simulink model "simulation_UMFCBF_"  (R2022a)
settings: Solver=VariableStepAuto  StartTime=0.0  StopTime=simTime  RelTol=1e-3
values from neighbouring files (symbols this model uses):
  a = 0.1    [setup_UMFCBF.m]
  delta = 2    [setup_UMFCBF.m]
  Icm = 1/2*m*robot_radius^2    (= 0.2385)    [setup_UMFCBF.m]
  Kd = 2.7    [setup_UMFCBF.m]
  Kp = 0.1    [setup_UMFCBF.m]
  m = 5.3    [setup_UMFCBF.m]
  obstacles = setup_environment(MAP,a,robot_radius)    [setup_UMFCBF.m]
  qg = [8 ; -3]    [setup_UMFCBF.m]
  qstart = [0 0 pi/2]'    [setup_UMFCBF.m]
  threshold_skip = 0    [setup_UMFCBF.m]
  vwstart = [0 0]'    [setup_UMFCBF.m]
libraries: slctrlblks x1
settings Model: Creator=mirkomizzoni  LastModifiedBy=dennis

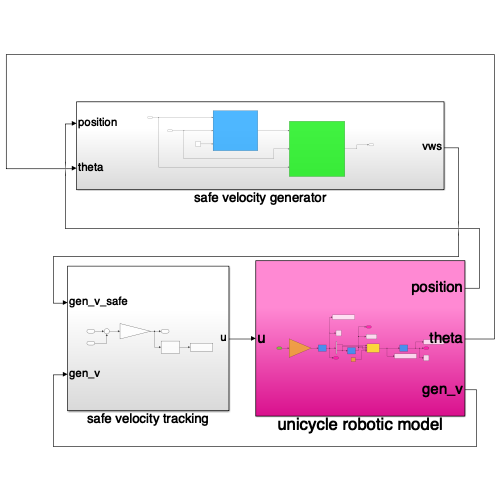
[thumbnail: Simulink's stored preview of the top-level diagram]
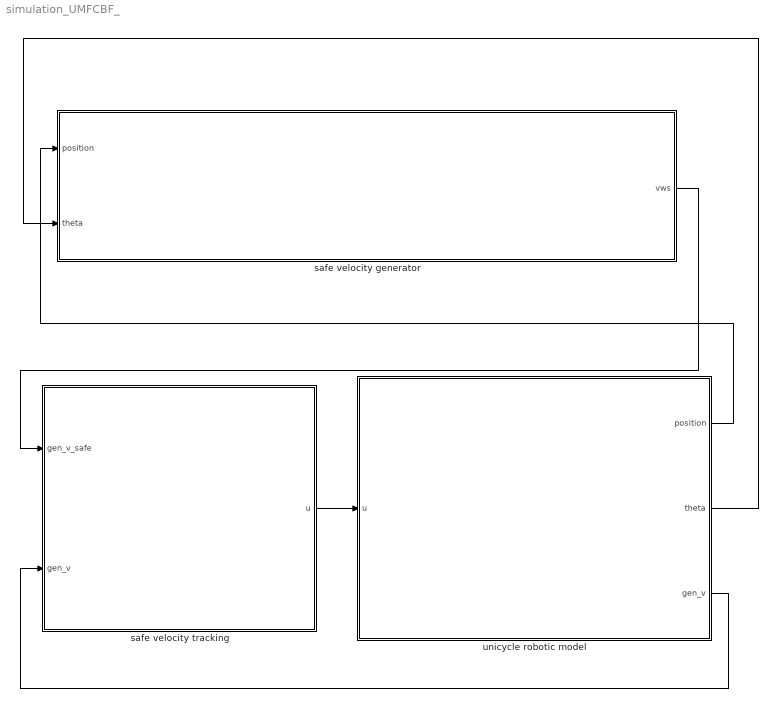
== system simulation_UMFCBF_ ==
  safe velocity generator : Subsystem
  safe velocity tracking : Subsystem
  unicycle robotic model : Subsystem
  wires:
  safe velocity generator/1(vws) -> safe velocity tracking/1(gen_v_safe)
  unicycle robotic model/3(gen_v) -> safe velocity tracking/2(gen_v)
  unicycle robotic model/1(position) -> safe velocity generator/1(position)
  unicycle robotic model/2(theta) -> safe velocity generator/2(theta)
  safe velocity tracking/1(u) -> unicycle robotic model/1(u)

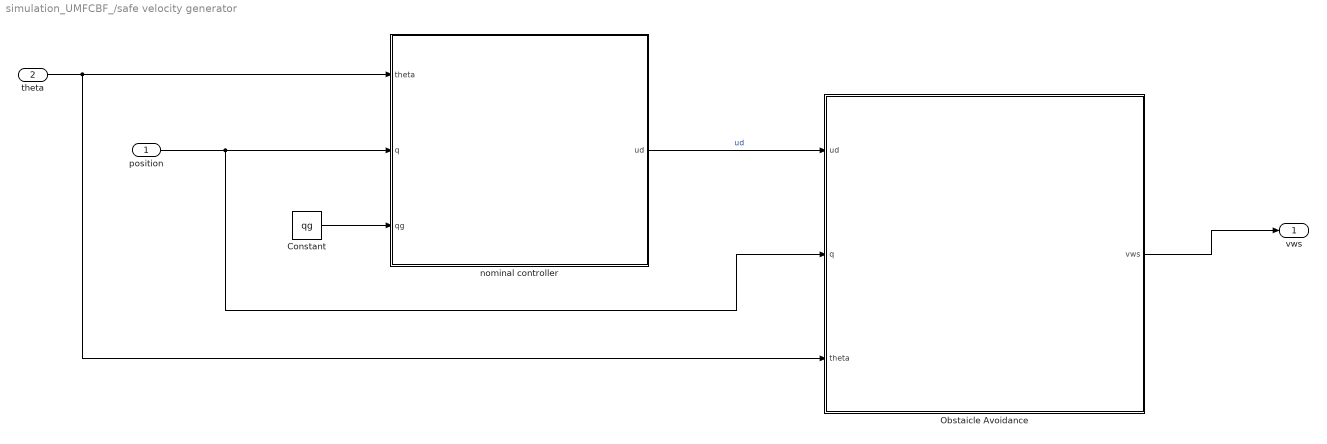
== system simulation_UMFCBF_/safe velocity generator ==
  position : Inport
  theta : Inport  Port=2
  Constant : Constant  Value=qg
  Obstaicle Avoidance : Subsystem
  nominal controller : Subsystem
  vws : Outport
  wires:
  Constant/1 -> nominal controller/3(qg)
  nominal controller/1(ud) -> Obstaicle Avoidance/1(ud)  "ud"
  Obstaicle Avoidance/1(vws) -> vws/1
  position/1 -> nominal controller/2(q), Obstaicle Avoidance/2(q)
  theta/1 -> Obstaicle Avoidance/3(theta), nominal controller/1(theta)

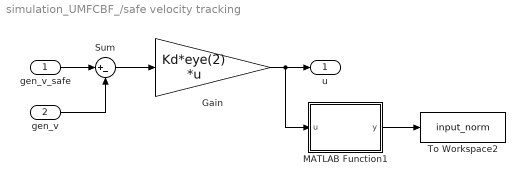
== system simulation_UMFCBF_/safe velocity tracking ==
  gen_v_safe : Inport
  gen_v : Inport  Port=2
  Gain : Gain  Gain=Kd*eye(2)  Multiplication=Matrix(K*u)
  MATLAB Function1 : MATLAB Function  TreatAsAtomicUnit=on
  Sum : Sum  Inputs=|+-
  To Workspace2 : ToWorkspace  VariableName=input_norm  SaveFormat=Timeseries  SampleTime=0.01
  u : Outport
  wires:
  Sum/1 -> Gain/1
  MATLAB Function1/1(y) -> To Workspace2/1
  gen_v_safe/1 -> Sum/1
  Gain/1 -> u/1, MATLAB Function1/1(u)
  gen_v/1 -> Sum/2

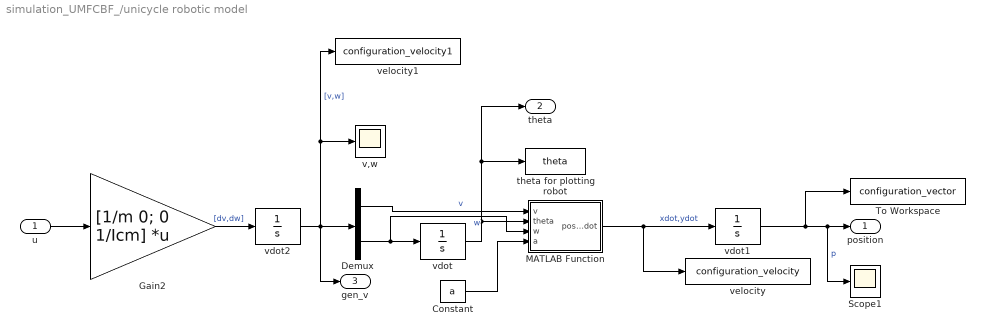
== system simulation_UMFCBF_/unicycle robotic model ==
  u : Inport
  Constant : Constant  Value=a
  Demux : Demux  Outputs=2
  Gain2 : Gain  Gain=[1/m 0; 0 1/Icm]  Multiplication=Matrix(K*u)
  MATLAB Function : MATLAB Function  TreatAsAtomicUnit=on
  Scope1 : Scope
  To Workspace : ToWorkspace  VariableName=configuration_vector  SaveFormat=Timeseries  SampleTime=0.01
  theta for plotting robot : ToWorkspace  VariableName=theta  SaveFormat=Timeseries  SampleTime=0.01
  v,w : Scope
  vdot : Integrator  InitialCondition=qstart(3)
  vdot1 : Integrator  InitialCondition=qstart(1:2)
  vdot2 : Integrator  InitialCondition=vwstart
  velocity : ToWorkspace  VariableName=configuration_velocity  SaveFormat=Timeseries  SampleTime=0.01
  velocity1 : ToWorkspace  VariableName=configuration_velocity1  SaveFormat=Timeseries  SampleTime=0.01
  position : Outport
  theta : Outport  Port=2
  gen_v : Outport  Port=3
  wires:
  vdot/1 -> theta/1, theta for plotting robot/1, MATLAB Function/2(theta)
  Demux/2 -> vdot/1, MATLAB Function/3(w)  "w"
  vdot2/1 -> gen_v/1, Demux/1, velocity1/1, v,w/1  "[v,w]"
  vdot1/1 -> position/1, Scope1/1, To Workspace/1  "p"
  Constant/1 -> MATLAB Function/4(a)
  MATLAB Function/1(positiondot) -> velocity/1, vdot1/1  "xdot,ydot"
  Gain2/1 -> vdot2/1  "[dv,dw]"
  Demux/1 -> MATLAB Function/1(v)  "v"
  u/1 -> Gain2/1

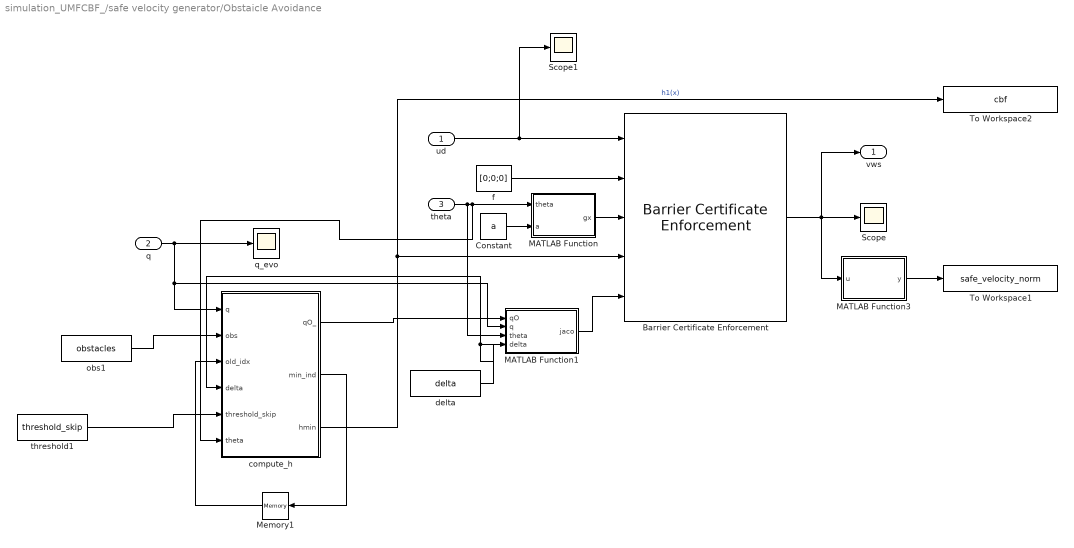
== system simulation_UMFCBF_/safe velocity generator/Obstaicle Avoidance ==
  ud : Inport
  q : Inport  Port=2
  theta : Inport  Port=3
  Barrier Certificate Enforcement : slctrlblks/Barrier Certificate Enforcement  nx=3  nu=2  nc=1  gamma=alpha  beta=1  external_umax=off  external_umin=off  Ts=0.01  maxiter=200  tol=1e-02  output_exitflag=off
      settings: SourceProductBaseCode=SD
  Constant : Constant  Value=a
  MATLAB Function : MATLAB Function  TreatAsAtomicUnit=on
  MATLAB Function1 : MATLAB Function  TreatAsAtomicUnit=on
  MATLAB Function3 : MATLAB Function  TreatAsAtomicUnit=on
  Memory1 : Memory  InitialCondition=1
  Scope : Scope
  Scope1 : Scope
  To Workspace1 : ToWorkspace  VariableName=safe_velocity_norm  SaveFormat=Timeseries  SampleTime=0.01
  To Workspace2 : ToWorkspace  VariableName=cbf  SaveFormat=Timeseries  SampleTime=0.01
  compute_h : MATLAB Function  TreatAsAtomicUnit=on
  delta : Constant  Value=delta  VectorParams1D=off
  f : Constant  Value=[0;0;0]  VectorParams1D=off
  obs1 : Constant  Value=obstacles  VectorParams1D=off
  q_evo : Scope
  threshold1 : Constant  Value=threshold_skip  VectorParams1D=off
  vws : Outport
  wires:
  q/1 -> q_evo/1, MATLAB Function1/2(q), compute_h/1(q)
  MATLAB Function3/1(y) -> To Workspace1/1
  f/1 -> Barrier Certificate Enforcement/2
  MATLAB Function1/1(jaco) -> Barrier Certificate Enforcement/5
  ud/1 -> Barrier Certificate Enforcement/1, Scope1/1
  Barrier Certificate Enforcement/1 -> MATLAB Function3/1(u), Scope/1, vws/1
  MATLAB Function/1(gx) -> Barrier Certificate Enforcement/3
  Constant/1 -> MATLAB Function/2(a)
  theta/1 -> MATLAB Function/1(theta), compute_h/6(theta), MATLAB Function1/3(theta)
  obs1/1 -> compute_h/2(obs)
  compute_h/2(min_ind) -> Memory1/1
  Memory1/1 -> compute_h/3(old_idx)
  threshold1/1 -> compute_h/5(threshold_skip)
  compute_h/3(hmin) -> To Workspace2/1, Barrier Certificate Enforcement/4  "h1(x)"
  compute_h/1(qO_) -> MATLAB Function1/1(qO)
  delta/1 -> MATLAB Function1/4(delta), compute_h/4(delta)

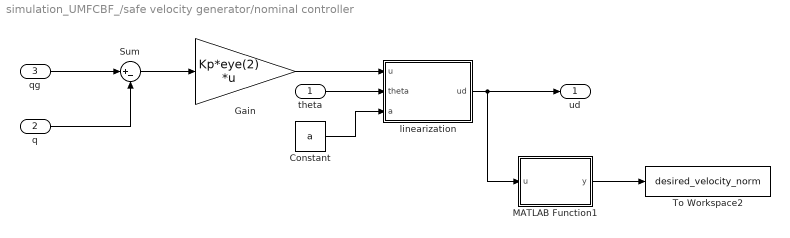
== system simulation_UMFCBF_/safe velocity generator/nominal controller ==
  theta : Inport
  q : Inport  Port=2
  qg : Inport  Port=3
  Constant : Constant  Value=a
  Gain : Gain  Gain=Kp*eye(2)  Multiplication=Matrix(K*u)
  MATLAB Function1 : MATLAB Function  TreatAsAtomicUnit=on
  Sum : Sum  Inputs=|+-
  To Workspace2 : ToWorkspace  VariableName=desired_velocity_norm  SaveFormat=Timeseries  SampleTime=0.01
  linearization : MATLAB Function  TreatAsAtomicUnit=on
  ud : Outport
  wires:
  MATLAB Function1/1(y) -> To Workspace2/1
  q/1 -> Sum/2
  qg/1 -> Sum/1
  Sum/1 -> Gain/1
  linearization/1(ud) -> ud/1, MATLAB Function1/1(u)
  Gain/1 -> linearization/1(u)
  theta/1 -> linearization/2(theta)
  Constant/1 -> linearization/3(a)

== matlab function simulation_UMFCBF_/safe velocity generator/Obstaicle Avoidance/compute_h ==
  data: qO_ output; min_ind output; hmin output; q input; obs input; old_idx input; delta input; threshold_skip input; theta input
function [qO_,min_ind,hmin] = min_dist(q, obs, old_idx, delta, threshold_skip,theta)
    [~,n] = size(obs);
    o1 = obs(:,1);
    min_ind = 1;
    hmin = hMin(q, o1,theta,delta);

    for i=2:n
        oi = obs(:,i);
        t = hMin(q, oi,theta,delta);
        if t<hmin
            min_ind = i;
            hmin = t;
        end
    end
%     oold = obs(:,old_idx);
%     old_dist = norm_obs(q,oold);
%     if abs(old_dist-min) < threshold_skip
%         min_ind = old_idx;
%         min = old_dist;
%     end
    qO = obs(:,min_ind);
    qO_ = qO(1:2);
end

function hmin = hMin(q, obs,theta,delta)
    d = norm(obs(1:2)-q(1:2));
    bear = atan2(obs(2)-q(2),obs(1)-q(1));
    hmin = d-obs(3)-obs(4)-delta*cos(theta-bear);
end

== matlab function simulation_UMFCBF_/safe velocity tracking/MATLAB Function1 ==
  data: u input; y output
function y = norm_func(u)
        
y = norm(u);

== matlab function simulation_UMFCBF_/safe velocity generator/Obstaicle Avoidance/MATLAB Function1 ==
  data: qO input; jaco output; q input; theta input; delta input
function jaco = jacob(qO,q,theta,delta)
   jac = (q-qO)'/norm(q-qO);
   jaco = [jac(1) jac(2) 0];
   ox = qO(1);
   oy = qO(2);
   x = q(1);
   y = q(2);
 
 
   jaco = [- (ox - x)/((ox - x)^2 + (oy - y)^2)^(1/2) - (delta*sin(theta - atan2(oy - y, ox - x))*(oy - y))/((ox - x)^2 + (oy - y)^2), - (oy - y)/((ox - x)^2 + (oy - y)^2)^(1/2) + (delta*sin(theta - atan2(oy - y, ox - x))*(ox - x))/((ox - x)^2 + (oy - y)^2), delta*sin(theta - atan2(oy - y, ox - x))];

end

== matlab function simulation_UMFCBF_/safe velocity generator/Obstaicle Avoidance/MATLAB Function3 ==
  data: u input; y output
function y = norm_func(u)
        
y = norm(u);

== matlab function simulation_UMFCBF_/safe velocity generator/nominal controller/MATLAB Function1 ==
  data: u input; y output
function y = norm_func(u)
        
y = norm(u);

== matlab function simulation_UMFCBF_/unicycle robotic model/MATLAB Function ==
  data: v input; positiondot output; theta input; w input; a input
function positiondot = posdot(v,theta,w,a)
        dx = v*cos(theta)-w*a*sin(theta);
        dy = v*sin(theta)+w*a*cos(theta);
        positiondot = [dx; dy];
end

== matlab function simulation_UMFCBF_/safe velocity generator/nominal controller/linearization ==
  data: u input; ud output; theta input; a input
function ud = transf_T(u, theta, a)
    Tm1 = [cos(theta) sin(theta); -sin(theta)/a cos(theta)/a];
    ud = Tm1*u;
end

== matlab function simulation_UMFCBF_/safe velocity generator/Obstaicle Avoidance/MATLAB Function ==
  data: theta input; gx output; a input
function gx = g(theta, a)
    gx = [cos(theta) -a*sin(theta); sin(theta) a*cos(theta); 0 1];
end
